simulink model "SingleCell"  (R2019a)
settings: Solver=VariableStepAuto  StartTime=0.0  StopTime=2355  RelTol=1e-3
values from neighbouring files (symbols this model uses):
  Q = 31.2    [workspace.mat]
undefined symbols (not defined in the file or in its folder): ocv, sigbuilder_block, soc
settings Model: Creator=sujan  LastModifiedBy=sujan

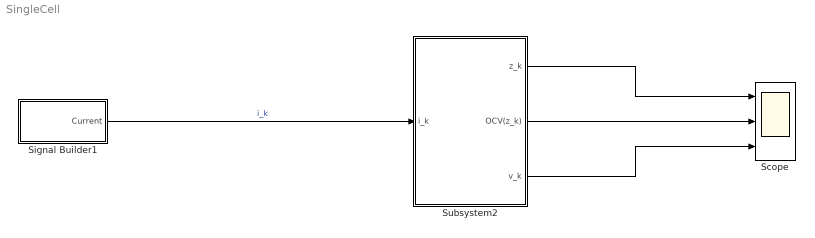
== system SingleCell ==
  Scope : Scope  NumInputPorts=3
  Signal Builder1 : Subsystem  Tag=STV Subsys  LoadFcn=sigbuilder_block('load');  StartFcn=sigbuilder_block('start');  StopFcn=sigbuilder_block('stop');  ClipboardFcn=sigbuilder_block('clipboard');  mask(Sigbuilder block){tuvar=[0:10]}
      mask help: Simulink:masks:SigbuilderBlock_MD
      mask init:
      | if ~strcmp(get_param(bdroot(gcbh),'SimulationStatus'),'stopped') tuvar = sigbuilder_block('maskInit'); end
      settings: CopyFcn=sigbuilder_block('copy');  DeleteFcn=sigbuilder_block('delete');  ModelCloseFcn=sigbuilder_block('modelClose');  PreSaveFcn=sigbuilder_block('preSave');  PauseFcn=sigbuilder_block('pause');  ContinueFcn=sigbuilder_block('continue');  NameChangeFcn=sigbuilder_block('namechange');  OpenFcn=sigbuilder_block('open',[339.6 151.8 550.8 400.2 ]);  CloseFcn=sigbuilder_block('close');
      mask Display: plot(0, 0, 100, 100,[2, 2, 32, 32, 2], [68, 8, 8, 68, 68],[32, 2], [38, 38], [32, 19, 2],[53, 60, 44], [32, 17, 17, 2],[16, 16, 31, 31]);txt = getActiveGroup(gcbh);text(2, 100, txt,'verticalAlignment', 'top');
  Subsystem2 : Subsystem
  wires:
  Subsystem2/1(z_k) -> Scope/1
  Subsystem2/2(OCV(z_k)) -> Scope/2
  Subsystem2/3(v_k) -> Scope/3
  Signal Builder1/1(Current) -> Subsystem2/1(i_k)  "i_k"

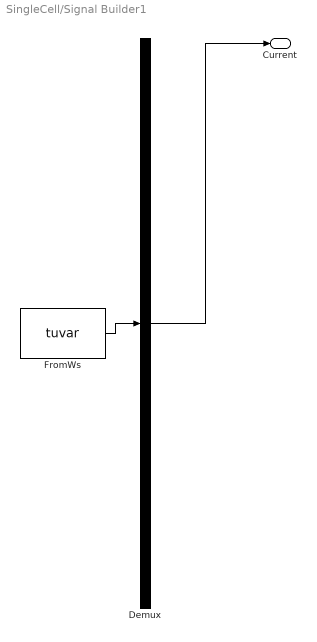
== system SingleCell/Signal Builder1 ==
  Demux : Demux  Tag=STV Demux  Outputs=1
  FromWs : FromWorkspace  Tag=STV FromWs  VariableName=tuvar  SampleTime=0
      SigBuilderData=|
      | common.afterFinalStr = 'Extrapolate'
      | common.sampleTime = 0
      | dataSet.timeRange = [0.0176671365608 124.786676059]
      | dataSet.name = 'Sheet1'
      | sbobj.Groups.Name = 'Sheet1'
      | sbobj.Groups.Signals.Name = 'Current'
      | sbobj.Groups.Signals.XData = [0.0176671365608 0.117667136561 0.219171291651 0.303787743842 0.378074200794 0.445155666779 0.506826698763 0.564234547563 0.618167124509 0.669194043835 0.717743348713 0.76414658576 ... (9908 elements, 1x9908)]
      | sbobj.Groups.Signals.YData = [12.5889164833 11.9192877182 11.9507289477 11.977007609 11.9982612876 12.017479777 12.0351748521 12.0516692795 12.0671847455 12.0818815279 12.095880078 12.1092736996 ... (9908 elements, 1x9908)]
      | sbobj.Groups.TimeRange = [0.0176671365608 124.786676059]
  Current : Outport  Tag=STV Outport
  wires:
  Demux/1 -> Current/1
  FromWs/1 -> Demux/1

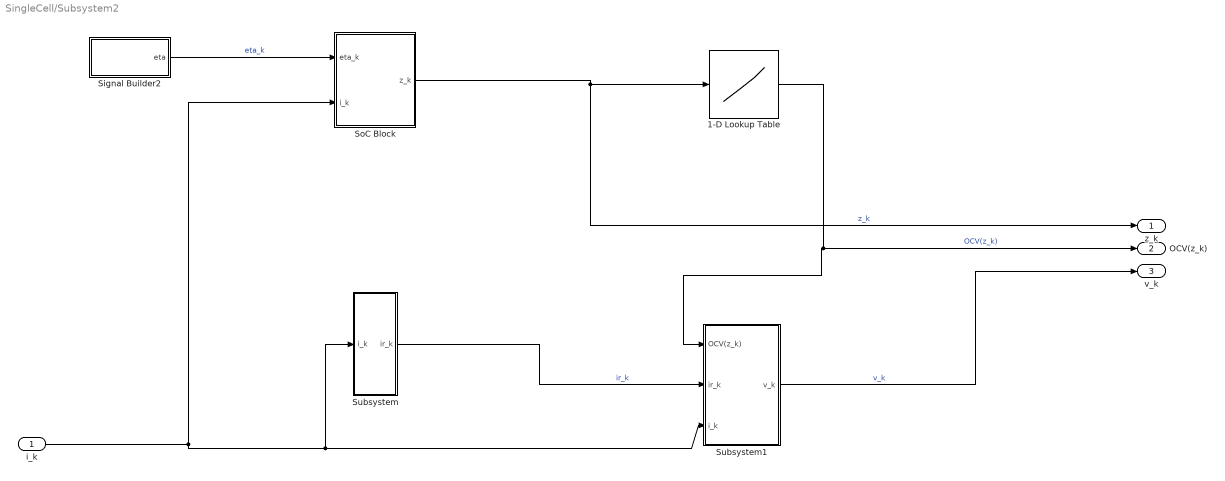
== system SingleCell/Subsystem2 ==
  i_k : Inport
  1-D Lookup Table : Lookup_n-D  NumberOfTableDimensions=1  LookupTableObject=Em  BreakpointsForDimension1=soc.soc  Table=ocv.ocv  InternalRulePriority=Speed  RndMeth=Simplest  InputSameDT=on
  Signal Builder2 : Subsystem  Tag=STV Subsys  LoadFcn=sigbuilder_block('load');  StartFcn=sigbuilder_block('start');  StopFcn=sigbuilder_block('stop');  ClipboardFcn=sigbuilder_block('clipboard');  mask(Sigbuilder block){tuvar=[0:10]}
      mask help: Simulink:masks:SigbuilderBlock_MD
      mask init:
      | if ~strcmp(get_param(bdroot(gcbh),'SimulationStatus'),'stopped') tuvar = sigbuilder_block('maskInit'); end
      settings: CopyFcn=sigbuilder_block('copy');  DeleteFcn=sigbuilder_block('delete');  ModelCloseFcn=sigbuilder_block('modelClose');  PreSaveFcn=sigbuilder_block('preSave');  PauseFcn=sigbuilder_block('pause');  ContinueFcn=sigbuilder_block('continue');  NameChangeFcn=sigbuilder_block('namechange');  OpenFcn=sigbuilder_block('open',[402.6 159.6 550.8 400.2 ]);  CloseFcn=sigbuilder_block('close');
      mask Display: plot(0, 0, 100, 100,[2, 2, 32, 32, 2], [68, 8, 8, 68, 68],[32, 2], [38, 38], [32, 19, 2],[53, 60, 44], [32, 17, 17, 2],[16, 16, 31, 31]);txt = getActiveGroup(gcbh);text(2, 100, txt,'verticalAlignment', 'top');
  "SoC Block " : Subsystem
  Subsystem : Subsystem
  Subsystem1 : Subsystem
  z_k : Outport
  OCV(z_k) : Outport  Port=2
  v_k : Outport  Port=3
  wires:
  1-D Lookup Table/1 -> Subsystem1/1(OCV(z_k)), OCV(z_k)/1  "OCV(z_k)"
  i_k/1 -> Subsystem/1(i_k), Subsystem1/3(i_k), "SoC Block "/2(i_k)
  Subsystem1/1(v_k) -> v_k/1  "v_k"
  "SoC Block "/1(z_k) -> z_k/1, 1-D Lookup Table/1  "z_k"
  Subsystem/1(ir_k) -> Subsystem1/2(ir_k)  "ir_k"
  Signal Builder2/1(eta) -> "SoC Block "/1(eta_k)  "eta_k"

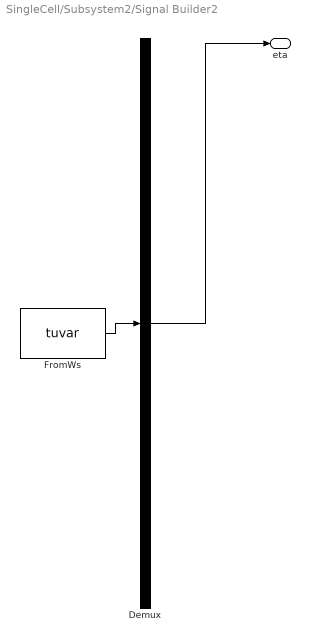
== system SingleCell/Subsystem2/Signal Builder2 ==
  Demux : Demux  Tag=STV Demux  Outputs=1
  FromWs : FromWorkspace  Tag=STV FromWs  VariableName=tuvar  SampleTime=0
      SigBuilderData=|
      | common.afterFinalStr = 'Extrapolate'
      | common.sampleTime = 0
      | dataSet.timeRange = [0.0176671365608 124.786676059]
      | dataSet.name = 'Sheet1'
      | sbobj.Groups.Name = 'Sheet1'
      | sbobj.Groups.Signals.Name = 'eta'
      | sbobj.Groups.Signals.XData = [0.0176671365608 0.117667136561 0.219171291651 0.303787743842 0.378074200794 0.445155666779 0.506826698763 0.564234547563 0.618167124509 0.669194043835 0.717743348713 0.76414658576 ... (9908 elements, 1x9908)]
      | sbobj.Groups.Signals.YData = [0.954687407395 0.903905741593 0.906290104529 0.908282961266 0.909894745679 0.911352190394 0.91269410615 0.913944970125 0.915121594024 0.916236132604 0.917297720353 0.918313433014 ... (9908 elements, 1x9908)]
      | sbobj.Groups.TimeRange = [0.0176671365608 124.786676059]
  eta : Outport  Tag=STV Outport
  wires:
  Demux/1 -> eta/1
  FromWs/1 -> Demux/1

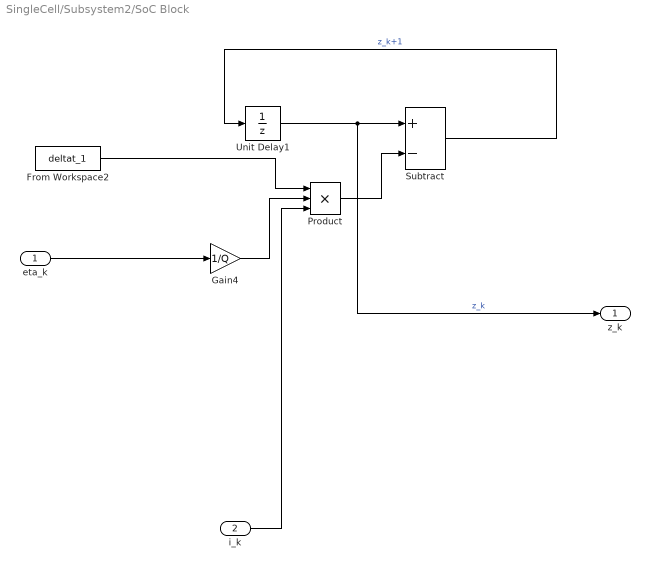
== system SingleCell/Subsystem2/SoC Block  ==
  eta_k : Inport
  i_k : Inport  Port=2
  From Workspace2 : FromWorkspace  VariableName=deltat_1  SampleTime=0
  Gain4 : Gain  Gain=1/Q
  Product : Product  Inputs=3
  Subtract : Sum  Inputs=+-
  Unit Delay1 : UnitDelay  InitialCondition=100  HasFrameUpgradeWarning=on
  z_k : Outport
  wires:
  Product/1 -> Subtract/2
  From Workspace2/1 -> Product/1
  Unit Delay1/1 -> z_k/1, Subtract/1  "z_k"
  eta_k/1 -> Gain4/1
  Gain4/1 -> Product/2
  i_k/1 -> Product/3
  Subtract/1 -> Unit Delay1/1  "z_k+1"

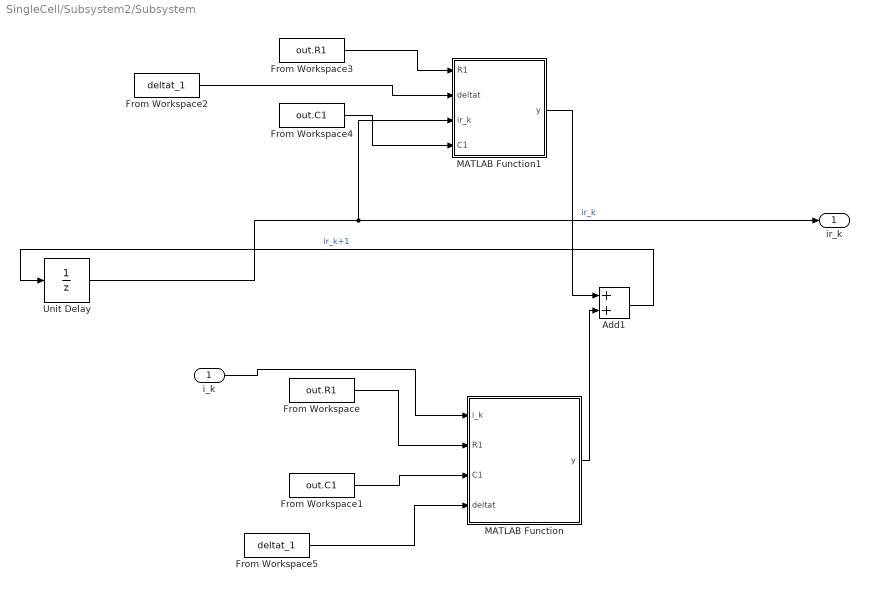
== system SingleCell/Subsystem2/Subsystem ==
  i_k : Inport
  Add1 : Sum
  From Workspace : FromWorkspace  VariableName=out.R1  SampleTime=0
  From Workspace1 : FromWorkspace  VariableName=out.C1  SampleTime=0
  From Workspace2 : FromWorkspace  VariableName=deltat_1  SampleTime=0
  From Workspace3 : FromWorkspace  VariableName=out.R1  SampleTime=0
  From Workspace4 : FromWorkspace  VariableName=out.C1  SampleTime=0
  From Workspace5 : FromWorkspace  VariableName=deltat_1  SampleTime=0
  MATLAB Function : MATLAB Function  TreatAsAtomicUnit=on
  MATLAB Function1 : MATLAB Function  TreatAsAtomicUnit=on
  Unit Delay : UnitDelay  HasFrameUpgradeWarning=on
  ir_k : Outport
  wires:
  MATLAB Function1/1(y) -> Add1/1
  Unit Delay/1 -> MATLAB Function1/3(ir_k), ir_k/1  "ir_k"
  Add1/1 -> Unit Delay/1  "ir_k+1"
  i_k/1 -> MATLAB Function/1(i_k)
  MATLAB Function/1(y) -> Add1/2
  From Workspace/1 -> MATLAB Function/2(R1)
  From Workspace4/1 -> MATLAB Function1/4(C1)
  From Workspace3/1 -> MATLAB Function1/1(R1)
  From Workspace1/1 -> MATLAB Function/3(C1)
  From Workspace2/1 -> MATLAB Function1/2(deltat)
  From Workspace5/1 -> MATLAB Function/4(deltat)

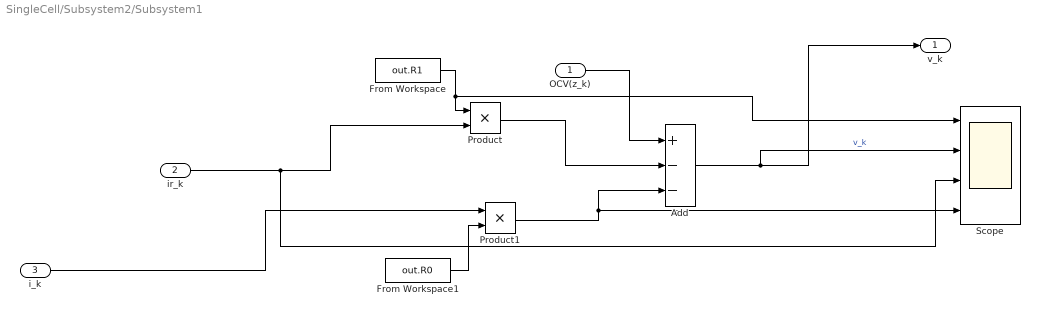
== system SingleCell/Subsystem2/Subsystem1 ==
  OCV(z_k) : Inport
  ir_k : Inport  Port=2
  i_k : Inport  Port=3
  Add : Sum  Inputs=+--
  From Workspace : FromWorkspace  VariableName=out.R1  SampleTime=0
  From Workspace1 : FromWorkspace  VariableName=out.R0  SampleTime=0
  Product : Product
  Product1 : Product
  Scope : Scope  NumInputPorts=4
  v_k : Outport
  wires:
  ir_k/1 -> Scope/3, Product/2
  Product/1 -> Add/2
  Product1/1 -> Scope/4, Add/3
  i_k/1 -> Product1/1
  OCV(z_k)/1 -> Add/1
  Add/1 -> Scope/2, v_k/1  "v_k"
  From Workspace1/1 -> Product1/2
  From Workspace/1 -> Scope/1, Product/1

== matlab function SingleCell/Subsystem2/Subsystem/MATLAB Function1 ==
  data: R1 input; deltat input; ir_k input; C1 input; y output
function y = fcn(R1,deltat, ir_k, C1)

y =ir_k*(exp(-deltat/(R1*C1)));

== matlab function SingleCell/Subsystem2/Subsystem/MATLAB Function ==
  data: i_k input; R1 input; C1 input; y output; deltat input
function y = fcn(i_k, R1,C1, deltat)

y = i_k*(1-exp(-deltat/(R1*C1)));
